simulink model "CodeGen_Cplus_solution"  (R2019b)
settings: Solver=VariableStepAuto  StartTime=0.0  StopTime=10  RelTol=1e-3  EnableMultiTasking=on
undefined symbols (not defined in the file): xc7k325tffg900
libraries: ModelComposer x3, visionsinks x3, Sobeledge_lib x2, dspvision x1
settings Model: Creator=dvancamp  LastModifiedBy=viswanad
settings DataIOCC: LimitDataPoints=on  ReturnWorkspaceOutputs=off
settings OptimizationCC: LifeSpan=inf
settings DebuggingCC: InheritedTsInSrcMsg=none  AllowSymbolicDim=off  SFUnexpectedBacktrackingDiag=warning  SFNoUnconditionalDefaultTransitionDiag=warning  ArithmeticOperatorsInVariantConditions=warning
settings ModelReferenceCC: PropagateSignalLabelsOutOfModel=off
settings SFSimCC: SimUseLocalCustomCode=off  CustomCodeUndefinedFunction=UseInterfaceOnly
settings RTWCC: RTWUseLocalCustomCode=off
settings CodeAppCC: StateflowObjectComments=on
settings GRTTargetCC: TargetLangStandard=C89/C90 (ANSI)
settings ConfigComp: CovMetricSettings=dw  CovHtmlReporting=on  CovSaveCumulativeToWorkspaceVar=on  CovSaveSingleToWorkspaceVar=on  CovExternalEMLEnable=off

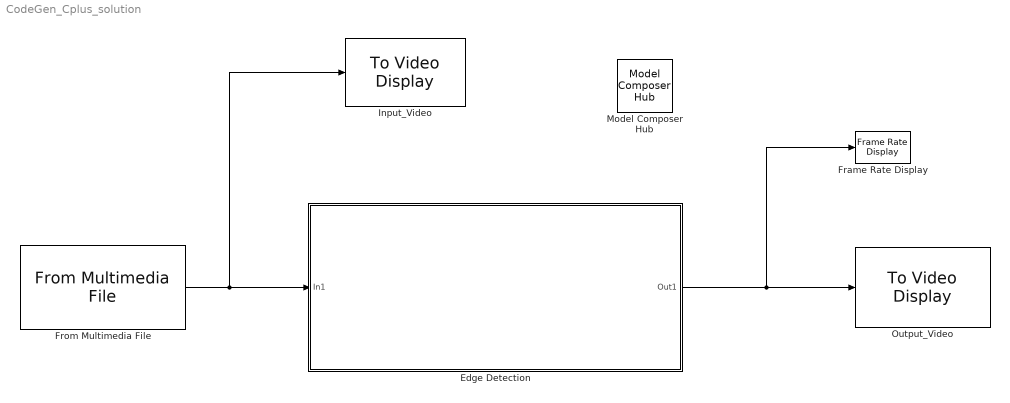
== system CodeGen_Cplus_solution ==
  Edge Detection : Subsystem
  Frame Rate Display : visionsinks/Frame Rate Display  UpdateRate=10
      settings: SourceProductName=Computer Vision Toolbox  SourceProductBaseCode=VP
  From Multimedia File : dspvision/From Multimedia File  inputFilename=visiontraffic.avi  readRange=[1 Inf]  loop=on  numPlays=inf  outputStreams=Video only  videoDataType=uint8  audioDataType=int16  inheritSampleTime=off  userDefinedSampleTime=1/30  noAudioOutput=off  isIntensityVideo=off  fourcc=Intensity  colorVideoFormat=Separate color signals  outputEOF=off  dataOrg=Column-major  audioFrameSize=1024  computeAudioFrameSize=off  outSamplingMode=Sample based
      settings: SourceProductName=DSP System Toolbox  SourceProductBaseCode=DS
  Input_Video : visionsinks/To Video Display  windowSizeMode=Normal  openAtMdlStart=on  fullScreen=off  videoWindowX=2068  videoWindowY=268  saveWindowSize=off  videoWindowWidth=581  videoWindowHeight=403  inputColorFormat=RGB  inputType=Obsolete  imagePorts=One multidimensional signal  OutputDevice=On-screen video monitor  dataOrg=Column-major  isWindowOpen=off
      settings: SourceProductName=Computer Vision Toolbox
  Model Composer Hub : ModelComposer/Model Composer Hub  Description=Performs multiplication  CodeGeneration=off  SubsystemName=Edge Detection  TargetDirectory=./codegen_edge_detection2  ExportType=HLS C++ code  IpVendor=xilinx.com  IpLibrary=hls  IpVersion=1.0  IpHWLanguage=Verilog  AieCompilerOptions={}  CreateTestbench=on  TestbenchStackSize=10  RunAieSim=off  AieSimTimeout=50000  LaunchVitisAnalyzer=off  RunX86Sim=on  X86SimTimeout=10  ProjDevice=Kintex-7 KC705 Evaluation Platform (xc7k325tffg900-2)  ProjDevicePart=xc7k325tffg900-2  SamplePeriod=-1  ClockFrequency=200  DataPathParallelism=1
  Output_Video : visionsinks/To Video Display  windowSizeMode=True size (1:1)  openAtMdlStart=on  fullScreen=off  videoWindowX=2667  videoWindowY=267  saveWindowSize=off  videoWindowWidth=640  videoWindowHeight=360  inputColorFormat=RGB  inputType=Obsolete  imagePorts=One multidimensional signal  OutputDevice=On-screen video monitor  dataOrg=Column-major  isWindowOpen=off
      settings: SourceProductName=Computer Vision Toolbox
  wires:
  From Multimedia File/1 -> Input_Video/1, Edge Detection/1(In1)
  Edge Detection/1(Out1) -> Frame Rate Display/1, Output_Video/1

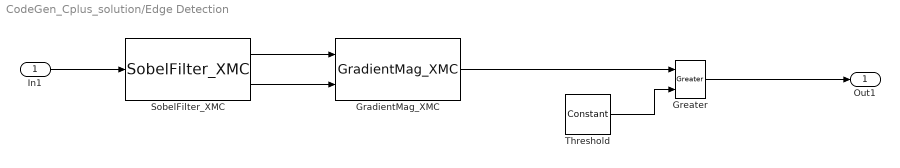
== system CodeGen_Cplus_solution/Edge Detection ==
  In1 : Inport
  GradientMag_XMC : Sobeledge_lib/GradientMag_XMC  LibraryFunction=GradientMag_XMC  IncludeFiles={'GradientMag_Wrap.h'}  SourceFiles={}  IncludeDirectories={'./include'}  TemplateParams={'int ROWS'; 'int COLS'; 'int NPC'}  FunctionParamTypes={xmcDataType('void'); xmcDataType('uint16_t'); xmcDataType('uint16_t'); xmcDataType('uint16_t'); xmcDataType('int')}  FunctionParamPassbys={0.000000000000000000e+00; 0.000000000000000000e+00; 0.000000000000000000e+00; 0.000000000000000000e+00; 0.000000000000000000e+00}  FunctionParamDimensions={'1'; '[ROWS][COLS]'; '[ROWS][COLS]'; '[ROWS][COLS]'; '1'}  FunctionParamNames={'return'; 'inX'; 'inY'; 'Out'; 'NPC'}  FunctionParamDir={0.000000000000000000e+00; 1.000000000000000000e+00; 1.000000000000000000e+00; 2.000000000000000000e+00; 3.000000000000000000e+00}  FunctionParamSupportsStreaming={true; true; true; true; true}  BufferDepth={'0'}  FunctionParamValues={'0'; '0'; '0'; '0'; '0'}  ThroughputFactors={''}  NPC=1
  Greater : ModelComposer/Greater  Description=Performs multiplication
  SobelFilter_XMC : Sobeledge_lib/SobelFilter_XMC  LibraryFunction=SobelFilter_XMC  IncludeFiles={'sobelfilter_Wrap.h'}  SourceFiles={}  IncludeDirectories={'./include'}  TemplateParams={'int ROWS'; 'int COLS'; 'int NPC'}  FunctionParamTypes={xmcDataType('void'); xmcDataType('uint8_t'); xmcDataType('uint16_t'); xmcDataType('uint16_t'); xmcDataType('int')}  FunctionParamPassbys={0.000000000000000000e+00; 0.000000000000000000e+00; 0.000000000000000000e+00; 0.000000000000000000e+00; 0.000000000000000000e+00}  FunctionParamDimensions={'1'; '[ROWS][COLS]'; '[ROWS][COLS]'; '[ROWS][COLS]'; '1'}  FunctionParamNames={'return'; 'in'; 'outX'; 'outY'; 'NPC'}  FunctionParamDir={0.000000000000000000e+00; 1.000000000000000000e+00; 2.000000000000000000e+00; 2.000000000000000000e+00; 3.000000000000000000e+00}  FunctionParamSupportsStreaming={true; true; true; true; true}  BufferDepth={'0'}  FunctionParamValues={'0'; '0'; '0'; '0'; '0'}  ThroughputFactors={''}  NPC=1
  Threshold : ModelComposer/Constant  Description=Performs multiplication  Value=150  VectorParams1D=off  SampleTime=-1  OutDataType=int16  TypeExp=''  Signedness=Signed  WordLength=16  FractionalLength=0  RoundingMode=Truncation to minus infinity  OverflowMode=Wrap around
  Out1 : Outport
  wires:
  In1/1 -> SobelFilter_XMC/1
  Threshold/1 -> Greater/2
  GradientMag_XMC/1 -> Greater/1
  SobelFilter_XMC/1 -> GradientMag_XMC/1
  SobelFilter_XMC/2 -> GradientMag_XMC/2
  Greater/1 -> Out1/1
